simulink subsystem "GS3DX_KD_Universal"  (R2025b)
settings: Solver=VariableStepAuto  StartTime=0.0  StopTime=10.0  RelTol=1e-3
model mask{StartPositionX=0, StartPositionY=0, StartVelocityX=0, StartVelocityY=0, DampeningX=0, DampeningY=0, RxPositionTargetPriority=None, RyPositionTargetPriority=None, RxVelocityTargetPriority=None, RyVelocityTargetPriority=None}
  mask prompts: StartPositionX "Initial Angle X (deg)"; StartPositionY "Initial Angle Y (deg)"; StartVelocityX "Initial Angular Velocity X (deg/s)"; StartVelocityY "Initial Angular Velocity Y (deg/s)"; DampeningX "Dampening X (Nm/deg/s)"; DampeningY "Dampening Y (Nm/deg/s)"; RxPositionTargetPriority "Position Target Priority X"; RyPositionTargetPriority "Position Target Priority Y"; RxVelocityTargetPriority "Velocity Target Priority X"; RyVelocityTargetPriority "Velocity Target Priority Y"
undefined symbols (not defined in the file): DampeningGlobalGain, LocalDampeningEnable
libraries: nesl_utility x19, fl_lib x6, sm_lib x3
settings Model: Creator=diete  LastModifiedBy=diete

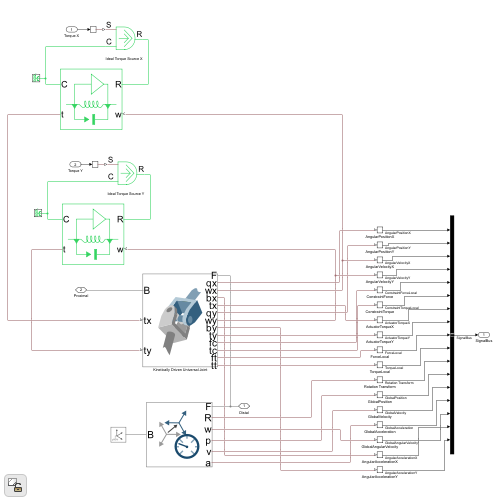
[thumbnail: Simulink's stored preview of the top-level diagram]
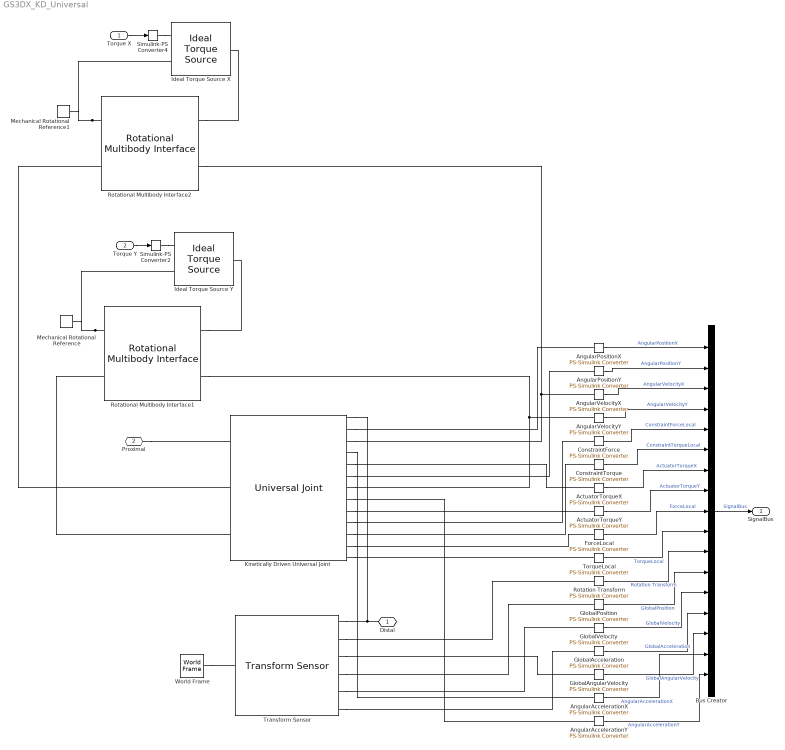
== system GS3DX_KD_Universal ==
  Torque X : Inport
  Torque Y : Inport  Port=2
  ActuatorTorqueX : nesl_utility/PS-Simulink Converter  PhysicalDomain=network_engine_domain  SubClassName=ps_output  LeftPortType=input  RightPortType=output  PseudoPeriodic=off  Frequencies=[]  VectorFormat=1-D array  Unit=inherit  AffineConversion=off
  ActuatorTorqueY : nesl_utility/PS-Simulink Converter  PhysicalDomain=network_engine_domain  SubClassName=ps_output  LeftPortType=input  RightPortType=output  PseudoPeriodic=off  Frequencies=[]  VectorFormat=1-D array  Unit=inherit  AffineConversion=off
  AngularAccelerationX : nesl_utility/PS-Simulink Converter  PhysicalDomain=network_engine_domain  SubClassName=ps_output  LeftPortType=input  RightPortType=output  PseudoPeriodic=off  Frequencies=[]  VectorFormat=1-D array  Unit=deg/s^2  AffineConversion=off
  AngularAccelerationY : nesl_utility/PS-Simulink Converter  PhysicalDomain=network_engine_domain  SubClassName=ps_output  LeftPortType=input  RightPortType=output  PseudoPeriodic=off  Frequencies=[]  VectorFormat=1-D array  Unit=deg/s^2  AffineConversion=off
  AngularPositionX : nesl_utility/PS-Simulink Converter  PhysicalDomain=network_engine_domain  SubClassName=ps_output  LeftPortType=input  RightPortType=output  PseudoPeriodic=off  Frequencies=[]  VectorFormat=1-D array  Unit=deg  AffineConversion=off
  AngularPositionY : nesl_utility/PS-Simulink Converter  PhysicalDomain=network_engine_domain  SubClassName=ps_output  LeftPortType=input  RightPortType=output  PseudoPeriodic=off  Frequencies=[]  VectorFormat=1-D array  Unit=deg  AffineConversion=off
  AngularVelocityX : nesl_utility/PS-Simulink Converter  PhysicalDomain=network_engine_domain  SubClassName=ps_output  LeftPortType=input  RightPortType=output  PseudoPeriodic=off  Frequencies=[]  VectorFormat=1-D array  Unit=deg/s  AffineConversion=off
  AngularVelocityY : nesl_utility/PS-Simulink Converter  PhysicalDomain=network_engine_domain  SubClassName=ps_output  LeftPortType=input  RightPortType=output  PseudoPeriodic=off  Frequencies=[]  VectorFormat=1-D array  Unit=deg/s  AffineConversion=off
  Bus Creator : BusCreator  Inputs=17
  ConstraintForce : nesl_utility/PS-Simulink Converter  PhysicalDomain=network_engine_domain  SubClassName=ps_output  LeftPortType=input  RightPortType=output  PseudoPeriodic=off  Frequencies=[]  VectorFormat=1-D array  Unit=inherit  AffineConversion=off
  ConstraintTorque : nesl_utility/PS-Simulink Converter  PhysicalDomain=network_engine_domain  SubClassName=ps_output  LeftPortType=input  RightPortType=output  PseudoPeriodic=off  Frequencies=[]  VectorFormat=1-D array  Unit=inherit  AffineConversion=off
  ForceLocal : nesl_utility/PS-Simulink Converter  PhysicalDomain=network_engine_domain  SubClassName=ps_output  LeftPortType=input  RightPortType=output  PseudoPeriodic=off  Frequencies=[]  VectorFormat=1-D array  Unit=inherit  AffineConversion=off
  GlobalAcceleration : nesl_utility/PS-Simulink Converter  PhysicalDomain=network_engine_domain  SubClassName=ps_output  LeftPortType=input  RightPortType=output  PseudoPeriodic=off  Frequencies=[]  VectorFormat=1-D array  Unit=inherit  AffineConversion=off
  GlobalAngularVelocity : nesl_utility/PS-Simulink Converter  PhysicalDomain=network_engine_domain  SubClassName=ps_output  LeftPortType=input  RightPortType=output  PseudoPeriodic=off  Frequencies=[]  VectorFormat=1-D array  Unit=deg/s  AffineConversion=off
  GlobalPosition : nesl_utility/PS-Simulink Converter  PhysicalDomain=network_engine_domain  SubClassName=ps_output  LeftPortType=input  RightPortType=output  PseudoPeriodic=off  Frequencies=[]  VectorFormat=1-D array  Unit=inherit  AffineConversion=off
  GlobalVelocity : nesl_utility/PS-Simulink Converter  PhysicalDomain=network_engine_domain  SubClassName=ps_output  LeftPortType=input  RightPortType=output  PseudoPeriodic=off  Frequencies=[]  VectorFormat=1-D array  Unit=inherit  AffineConversion=off
  Ideal Torque Source X : fl_lib/Mechanical/Mechanical Sources/Ideal Torque Source
  Ideal Torque Source Y : fl_lib/Mechanical/Mechanical Sources/Ideal Torque Source
  Kinetically Driven Universal Joint : sm_lib/Joints/Universal Joint  JointMode=Normal  CompositeWrenchDir=BaseOnFollower  CompositeWrenchFrame=FollowerFrame  SenseConstraintForce=on  SenseConstraintTorque=on  SenseTotalForce=on  SenseTotalTorque=on  RxPositionTargetSpecify=off  RxPositionTargetPriority=High  RxPositionTargetValue=StartPositionX  RxPositionTargetValueUnits=deg  RxVelocityTargetSpecify=off  RxVelocityTargetPriority=High  RxVelocityTargetValue=StartVelocityX  RxVelocityTargetValueUnits=deg/s  RxEquilibriumPosition=0  RxEquilibriumPositionUnits=deg  RxSpringStiffness=0  RxSpringStiffnessUnits=N*m/deg  RxDampingCoefficient=DampeningX*LocalDampeningEnable*DampeningGlobalGain  RxDampingCoefficientUnits=N*m/(deg/s)  RxLowerLimitSpecify=off  RxLowerLimitBound=-120  RxLowerLimitBoundUnits=deg  RxLowerLimitStiffness=300  RxLowerLimitStiffnessUnits=N*m/deg  RxLowerLimitDamping=10  RxLowerLimitDampingUnits=N*m/(deg/s)  RxLowerLimitTransitionRegionWidth=0.1  RxLowerLimitTransitionRegionWidthUnits=deg  RxUpperLimitSpecify=off  RxUpperLimitBound=0  RxUpperLimitBoundUnits=deg  RxUpperLimitStiffness=300  RxUpperLimitStiffnessUnits=N*m/deg  RxUpperLimitDamping=10  RxUpperLimitDampingUnits=N*m/(deg/s)  RxUpperLimitTransitionRegionWidth=0.1  RxUpperLimitTransitionRegionWidthUnits=deg  RxTorqueActuationMode=InputTorque  RxMotionActuationMode=ComputedMotion  RxSensePosition=on  RxSenseVelocity=on  RxSenseAcceleration=on  RxSenseTorqueForce=on  RxSenseLowerLimitTorqueForce=off  RxSenseUpperLimitTorqueForce=off  RyPositionTargetSpecify=off  RyPositionTargetPriority=Low  RyPositionTargetValue=StartPositionY  RyPositionTargetValueUnits=deg  RyVelocityTargetSpecify=off  RyVelocityTargetPriority=Low  RyVelocityTargetValue=StartVelocityY  RyVelocityTargetValueUnits=deg/s  RyEquilibriumPosition=0  RyEquilibriumPositionUnits=deg  RySpringStiffness=0  RySpringStiffnessUnits=N*m/deg  RyDampingCoefficient=DampeningY*LocalDampeningEnable*DampeningGlobalGain  RyDampingCoefficientUnits=N*m/(deg/s)  RyLowerLimitSpecify=off  RyLowerLimitBound=-30  RyLowerLimitBoundUnits=deg  RyLowerLimitStiffness=300  RyLowerLimitStiffnessUnits=N*m/deg  RyLowerLimitDamping=10  RyLowerLimitDampingUnits=N*m/(deg/s)  RyLowerLimitTransitionRegionWidth=0.1  RyLowerLimitTransitionRegionWidthUnits=deg  RyUpperLimitSpecify=off  RyUpperLimitBound=30  RyUpperLimitBoundUnits=deg  RyUpperLimitStiffness=300  RyUpperLimitStiffnessUnits=N*m/deg  RyUpperLimitDamping=10  RyUpperLimitDampingUnits=N*m/(deg/s)  RyUpperLimitTransitionRegionWidth=0.1  RyUpperLimitTransitionRegionWidthUnits=deg  RyTorqueActuationMode=InputTorque  RyMotionActuationMode=ComputedMotion  RySensePosition=on  RySenseVelocity=on  RySenseAcceleration=on  RySenseTorqueForce=on  RySenseLowerLimitTorqueForce=off  RySenseUpperLimitTorqueForce=off
  Mechanical Rotational Reference : fl_lib/Mechanical/Rotational Elements/Mechanical Rotational Reference
  Mechanical Rotational Reference1 : fl_lib/Mechanical/Rotational Elements/Mechanical Rotational Reference
  Rotation Transform : nesl_utility/PS-Simulink Converter  PhysicalDomain=network_engine_domain  SubClassName=ps_output  LeftPortType=input  RightPortType=output  PseudoPeriodic=off  Frequencies=[]  VectorFormat=1-D array  Unit=inherit  AffineConversion=off
  Rotational Multibody Interface1 : fl_lib/Mechanical/Multibody Interfaces/Rotational Multibody Interface
  Rotational Multibody Interface2 : fl_lib/Mechanical/Multibody Interfaces/Rotational Multibody Interface
  Simulink-PS Converter2 : nesl_utility/Simulink-PS Converter  PhysicalDomain=network_engine_domain  SubClassName=ps_input  LeftPortType=input  RightPortType=output  PseudoPeriodic=off  Frequencies=[]  NoiseDistribution=none  NoiseParameters=[]  Unit=1  AffineConversion=off  FilteringAndDerivatives=provide  SimscapeFilterOrder=1  InputFilterTimeConstant=0.001  UdotUserProvided=0
  Simulink-PS Converter4 : nesl_utility/Simulink-PS Converter  PhysicalDomain=network_engine_domain  SubClassName=ps_input  LeftPortType=input  RightPortType=output  PseudoPeriodic=off  Frequencies=[]  NoiseDistribution=none  NoiseParameters=[]  Unit=1  AffineConversion=off  FilteringAndDerivatives=provide  SimscapeFilterOrder=1  InputFilterTimeConstant=0.001  UdotUserProvided=0
  TorqueLocal : nesl_utility/PS-Simulink Converter  PhysicalDomain=network_engine_domain  SubClassName=ps_output  LeftPortType=input  RightPortType=output  PseudoPeriodic=off  Frequencies=[]  VectorFormat=1-D array  Unit=inherit  AffineConversion=off
  Transform Sensor : sm_lib/Frames and Transforms/Transform Sensor  MeasurementFrame=World  RotationSequence=XYX  SenseAngle=off  SenseAxis=off  SenseQ=off  SenseR=on  SenseRotationSequence=off  SenseOmegaX=off  SenseOmegaY=off  SenseOmegaZ=off  SenseOmega=on  SenseQDot=off  SenseRDot=off  SenseRotationSequenceDot=off  SenseAlphaX=off  SenseAlphaY=off  SenseAlphaZ=off  SenseAlpha=off  SenseQDDot=off  SenseRDDot=off  SenseX=off  SenseY=off  SenseZ=off  SenseXYZ=on  SenseRad=off  SenseAzim=off  SenseDist=off  SenseInc=off  SenseXDot=off  SenseYDot=off  SenseZDot=off  SenseXYZDot=on  SenseRadDot=off  SenseAzimDot=off  SenseDistDot=off  SenseIncDot=off  SenseXDDot=off  SenseYDDot=off  SenseZDDot=off  SenseXYZDDot=on  SenseRadDDot=off  SenseAzimDDot=off  SenseDistDDot=off  SenseIncDDot=off
  World Frame : sm_lib/Frames and Transforms/World Frame
  Distal : PMIOPort  Side=Right
  Proximal : PMIOPort  Port=2  Side=Left
  SignalBus : Outport
  wires:
  Bus Creator/1 -> SignalBus/1  "SignalBus"
  AngularVelocityY/1 -> Bus Creator/4  "AngularVelocityY"
  GlobalVelocity/1 -> Bus Creator/13  "GlobalVelocity"
  TorqueLocal/1 -> Bus Creator/10  "TorqueLocal"
  GlobalAngularVelocity/1 -> Bus Creator/15  "GlobalAngularVelocity"
  AngularPositionX/1 -> Bus Creator/1  "AngularPositionX"
  Rotation Transform/1 -> Bus Creator/11  "Rotation Transform"
  ForceLocal/1 -> Bus Creator/9  "ForceLocal"
  GlobalPosition/1 -> Bus Creator/12  "GlobalPosition"
  ConstraintTorque/1 -> Bus Creator/6  "ConstraintTorqueLocal"
  ConstraintForce/1 -> Bus Creator/5  "ConstraintForceLocal"
  GlobalAcceleration/1 -> Bus Creator/14  "GlobalAcceleration"
  Torque X/1 -> Simulink-PS Converter4/1
  Torque Y/1 -> Simulink-PS Converter2/1
  AngularVelocityX/1 -> Bus Creator/3  "AngularVelocityX"
  AngularPositionY/1 -> Bus Creator/2  "AngularPositionY"
  ActuatorTorqueX/1 -> Bus Creator/7  "ActuatorTorqueX"
  ActuatorTorqueY/1 -> Bus Creator/8  "ActuatorTorqueY"
  AngularAccelerationX/1 -> Bus Creator/16  "AngularAccelerationX"
  AngularAccelerationY/1 -> Bus Creator/17  "AngularAccelerationY"
  connections:
  Distal/RConn1 -- Transform Sensor/RConn1 -- Kinetically Driven Universal Joint/RConn1
  Rotational Multibody Interface1/LConn2 -- Ideal Torque Source Y/RConn2 -- Mechanical Rotational Reference/LConn1
  Rotational Multibody Interface2/LConn2 -- Ideal Torque Source X/RConn2 -- Mechanical Rotational Reference1/LConn1
  Rotational Multibody Interface2/RConn1 -- Kinetically Driven Universal Joint/RConn3 -- AngularVelocityX/LConn1
  Rotational Multibody Interface1/RConn1 -- Kinetically Driven Universal Joint/RConn7 -- AngularVelocityY/LConn1
  Transform Sensor/RConn3 -- GlobalAngularVelocity/LConn1
  Transform Sensor/RConn6 -- GlobalAcceleration/LConn1
  Transform Sensor/RConn2 -- Rotation Transform/LConn1
  World Frame/RConn1 -- Transform Sensor/LConn1
  Proximal/RConn1 -- Kinetically Driven Universal Joint/LConn1
  Transform Sensor/RConn4 -- GlobalPosition/LConn1
  Transform Sensor/RConn5 -- GlobalVelocity/LConn1
  Rotational Multibody Interface1/RConn2 -- Ideal Torque Source Y/LConn1
  Simulink-PS Converter2/RConn1 -- Ideal Torque Source Y/RConn1
  Rotational Multibody Interface2/RConn2 -- Ideal Torque Source X/LConn1
  Simulink-PS Converter4/RConn1 -- Ideal Torque Source X/RConn1
  Rotational Multibody Interface1/LConn1 -- Kinetically Driven Universal Joint/LConn3
  Rotational Multibody Interface2/LConn1 -- Kinetically Driven Universal Joint/LConn2
  Kinetically Driven Universal Joint/RConn12 -- ForceLocal/LConn1
  Kinetically Driven Universal Joint/RConn13 -- TorqueLocal/LConn1
  Kinetically Driven Universal Joint/RConn10 -- ConstraintForce/LConn1
  Kinetically Driven Universal Joint/RConn11 -- ConstraintTorque/LConn1
  Kinetically Driven Universal Joint/RConn2 -- AngularPositionX/LConn1
  Kinetically Driven Universal Joint/RConn6 -- AngularPositionY/LConn1
  Kinetically Driven Universal Joint/RConn5 -- ActuatorTorqueX/LConn1
  Kinetically Driven Universal Joint/RConn9 -- ActuatorTorqueY/LConn1
  Kinetically Driven Universal Joint/RConn4 -- AngularAccelerationX/LConn1
  Kinetically Driven Universal Joint/RConn8 -- AngularAccelerationY/LConn1
